simulink model "AWFG_concept_Phase1"  (R2018a)
settings: Solver=ode3  StartTime=0.0  StopTime=0.1  RelTol=1e-3  EnableMultiTasking=on
libraries: simulink x7
Description:
  | AWFG_concept: This model explores the implementation concept
  | of an arbitrary waveform generator (AWFG) in a real-time target
  | platform with a combination of CPU and FPGA code.
  | This concepts aims at minimizing changes in the FPGA programming.
settings Model: Creator=Estra  LastModifiedBy=Talha Rao
settings DataIOCC: LimitDataPoints=on  SaveFormat=Array
settings OptimizationCC: DefaultParameterBehavior=Inlined  UseDivisionForNetSlopeComputation=on  UseFloatMulNetSlope=on  InlineInvariantSignals=on  PassReuseOutputArgsAs=Individual arguments  ExpressionDepthLimit=2147483647  ZeroExternalMemoryAtStartup=off  ZeroInternalMemoryAtStartup=off  NoFixptDivByZeroProtection=on  EfficientFloat2IntCast=on  LifeSpan=1
settings DebuggingCC: SignalInfNanChecking=warning  UnderspecifiedInitializationDetection=Classic  MergeDetectMultiDrivingBlocksExec=none  SolverPrmCheckMsg=warning  ParameterTunabilityLossMsg=error  UniqueDataStoreMsg=warning  AllowSymbolicDim=off  StateNameClashWarn=warning  SFUnexpectedBacktrackingDiag=warning  SFNoUnconditionalDefaultTransitionDiag=warning  SFExecutionAtInitializationDiag=none
settings HardwareCC: ProdLongLongMode=on
settings ModelReferenceCC: PropagateSignalLabelsOutOfModel=off
settings SFSimCC: MATLABDynamicMemAlloc=off
settings RTWCC: SystemTargetFile=ert.tlc  TemplateMakefile=ert_default_tmf  GenerateReport=on  IncludeHyperlinkInReport=on  LaunchReport=on  GenerateTraceInfo=on  GenerateTraceReport=on  GenerateTraceReportSl=on  GenerateTraceReportSf=on  GenerateTraceReportEml=on  GenerateCodeMetricsReport=on
settings CodeAppCC: ForceParamTrailComments=on  IgnoreCustomStorageClasses=off  OperatorAnnotations=on  SimulinkDataObjDesc=on  SFDataObjDesc=on  CustomSymbolStrGlobalVar=rt$N$M  CustomSymbolStrType=$N$M  CustomSymbolStrFcn=$N$M$F  CustomSymbolStrMacro=$N$M  InsertBlockDesc=on  StateflowObjectComments=on
settings ERTTargetCC: GenerateSampleERTMain=on  IncludeMdlTerminateFcn=off  CombineSignalStateStructs=on  SupportAbsoluteTime=off  SupportComplex=off  SupportNonInlinedSFcns=on  InlinedParameterPlacement=NonHierarchical  ERTCustomFileTemplate=example_file_process.tlc  ERTFilePackagingFormat=CompactWithDataFile
settings ConfigComp: CovMetricSettings=dw  CovHtmlReporting=on  CovSaveCumulativeToWorkspaceVar=on  CovSaveSingleToWorkspaceVar=on  CovExternalEMLEnable=off

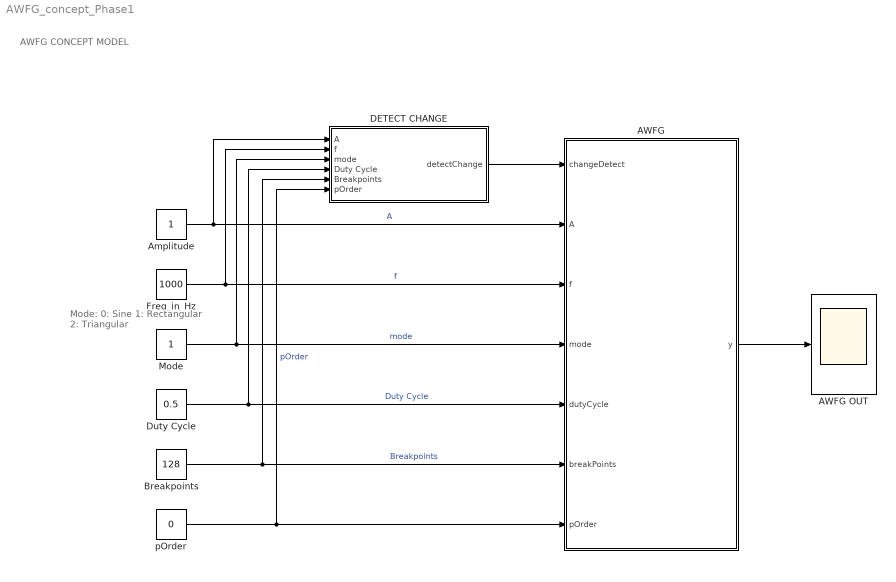
== system AWFG_concept_Phase1 ==
  note: AWFG CONCEPT MODEL
  note: Mode:
      | 0: Sine
      | 1: Rectangular
      | 2: Triangular
  AWFG : Subsystem
  AWFG OUT : Scope
  Amplitude : Constant
  Breakpoints : Constant  Value=128
  DETECT CHANGE : Subsystem
  Duty Cycle : Constant  Value=0.5
  Freq_in_Hz : Constant  Value=1000
  Mode : Constant
  pOrder : Constant  Value=0
  wires:
  AWFG/1(y) -> AWFG OUT/1
  DETECT CHANGE/1(detectChange) -> AWFG/1(changeDetect)
  Amplitude/1 -> DETECT CHANGE/1(A), AWFG/2(A)  "A"
  Freq_in_Hz/1 -> DETECT CHANGE/2(f), AWFG/3(f)  "f"
  Mode/1 -> DETECT CHANGE/3(mode), AWFG/4(mode)  "mode"
  Duty Cycle/1 -> DETECT CHANGE/4(Duty Cycle), AWFG/5(dutyCycle)  "Duty Cycle"
  Breakpoints/1 -> DETECT CHANGE/5(Breakpoints), AWFG/6(breakPoints)  "Breakpoints"
  pOrder/1 -> DETECT CHANGE/6(pOrder), AWFG/7(pOrder)  "pOrder"

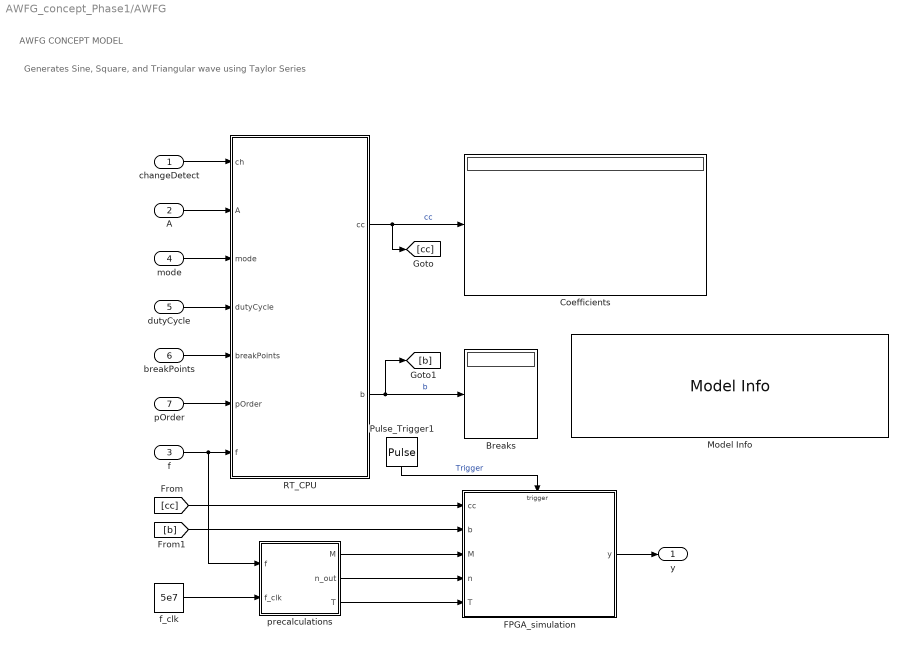
== system AWFG_concept_Phase1/AWFG ==
  note: Generates Sine, Square, and Triangular wave using Taylor Series
  note: AWFG CONCEPT MODEL
  changeDetect : Inport
  A : Inport  Port=2
  f : Inport  Port=3
  mode : Inport  Port=4
  dutyCycle : Inport  Port=5
  breakPoints : Inport  Port=6
  pOrder : Inport  Port=7
  Breaks : Display
  Coefficients : Display
  FPGA_simulation : Subsystem
  Model Info : simulink/Model-Wide Utilities/Model Info  Frame=on  DisplayStringWithTags=|  HorizontalTextAlignment=Left  LeftAlignmentValue=0.02
      | Model Info
      | Creator:       R. Estrada, FH JOANNEUM, 2018
      | Modified by: %<ModifiedBy>
      | Modify Date: %<ModifiedDate>
      | Version:%<ModelVersion>
      | Description:
      | %<Description>
  Pulse_Trigger1 : DiscretePulseGenerator  PulseType=Time based  Period=1/5e7  PulseWidth=50
  RT_CPU : MATLAB Function  TreatAsAtomicUnit=on
  f_clk : Constant  Value=5e7
  precalculations : Subsystem
  y : Outport
  wires:
  RT_CPU/2(b) -> [b], Breaks/1  "b"
  f_clk/1 -> precalculations/2(f_clk)
  RT_CPU/1(cc) -> Coefficients/1, [cc]  "cc"
  mode/1 -> RT_CPU/3(mode)
  f/1 -> precalculations/1(f), RT_CPU/7(f)
  breakPoints/1 -> RT_CPU/5(breakPoints)
  precalculations/2(n_out) -> FPGA_simulation/4(n)
  Pulse_Trigger1/1 -> FPGA_simulation/Trigger  "Trigger"
  precalculations/1(M) -> FPGA_simulation/3(M)
  precalculations/3(T) -> FPGA_simulation/5(T)
  FPGA_simulation/1(y) -> y/1
  A/1 -> RT_CPU/2(A)
  pOrder/1 -> RT_CPU/6(pOrder)
  dutyCycle/1 -> RT_CPU/4(dutyCycle)
  changeDetect/1 -> RT_CPU/1(ch)
  [b] -> FPGA_simulation/2(b)
  [cc] -> FPGA_simulation/1(cc)

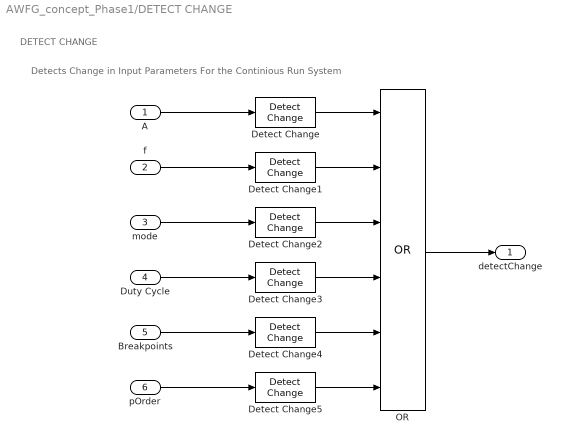
== system AWFG_concept_Phase1/DETECT CHANGE ==
  note: Detects Change in Input Parameters For the Continious Run System
  note: DETECT CHANGE
  A : Inport
  f : Inport  Port=2
  mode : Inport  Port=3
  Duty Cycle : Inport  Port=4
  Breakpoints : Inport  Port=5
  pOrder : Inport  Port=6
  Detect Change{,1..5} (6 alike) : simulink/Logic and Bit Operations/Detect Change  vinit=0  OutDataTypeStr=boolean
  OR : Logic  Operator=OR  Inputs=6  AllPortsSameDT=off  OutDataTypeStr=boolean
  detectChange : Outport
  wires:
  Detect Change3/1 -> OR/4
  mode/1 -> Detect Change2/1
  Detect Change5/1 -> OR/6
  Detect Change1/1 -> OR/2
  Breakpoints/1 -> Detect Change4/1
  pOrder/1 -> Detect Change5/1
  Detect Change4/1 -> OR/5
  Detect Change2/1 -> OR/3
  Detect Change/1 -> OR/1
  Duty Cycle/1 -> Detect Change3/1
  f/1 -> Detect Change1/1
  A/1 -> Detect Change/1
  OR/1 -> detectChange/1

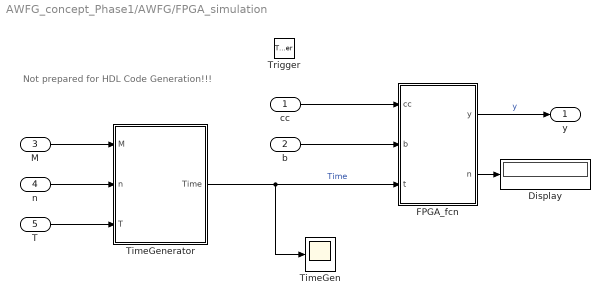
== system AWFG_concept_Phase1/AWFG/FPGA_simulation ==
  note: Not prepared for HDL Code Generation!!!
  cc : Inport
  b : Inport  Port=2
  M : Inport  Port=3
  n : Inport  Port=4
  T : Inport  Port=5
  Trigger : TriggerPort  VariantControl=(inherit)  PortDimensions=1
  Display : Display
  FPGA_fcn : MATLAB Function  TreatAsAtomicUnit=on
  TimeGen : Scope
  TimeGenerator : Subsystem
  y : Outport
  wires:
  T/1 -> TimeGenerator/3(T)
  n/1 -> TimeGenerator/2(n)
  cc/1 -> FPGA_fcn/1(cc)
  M/1 -> TimeGenerator/1(M)
  TimeGenerator/1(Time) -> FPGA_fcn/3(t), TimeGen/1  "Time"
  FPGA_fcn/1(y) -> y/1  "y"
  b/1 -> FPGA_fcn/2(b)
  FPGA_fcn/2(n) -> Display/1

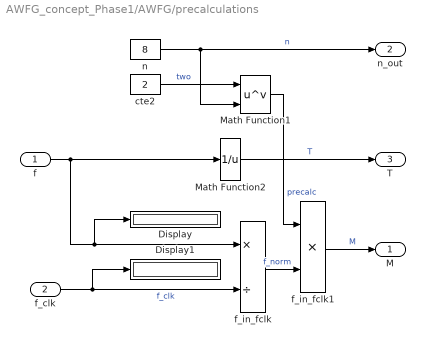
== system AWFG_concept_Phase1/AWFG/precalculations ==
  f : Inport
  f_clk : Inport  Port=2
  Display : Display
  Display1 : Display
  Math Function1 : Math  Operator=pow  SaturateOnIntegerOverflow=on
  Math Function2 : Math  Operator=reciprocal  SaturateOnIntegerOverflow=on
  cte2 : Constant  Value=2  SampleTime=-1
  f_in_fclk : Product  Inputs=*/
  f_in_fclk1 : Product  Inputs=**
  n : Constant  Value=8  SampleTime=-1
  M : Outport
  n_out : Outport  Port=2
  T : Outport  Port=3
  wires:
  cte2/1 -> Math Function1/1  "two"
  n/1 -> Math Function1/2, n_out/1  "n"
  Math Function1/1 -> f_in_fclk1/1  "precalc"
  Math Function2/1 -> T/1  "T"
  f_in_fclk1/1 -> M/1  "M"
  f_clk/1 -> f_in_fclk/2, Display1/1  "f_clk"
  f_in_fclk/1 -> f_in_fclk1/2  "f_norm"
  f/1 -> Math Function2/1, Display/1, f_in_fclk/1

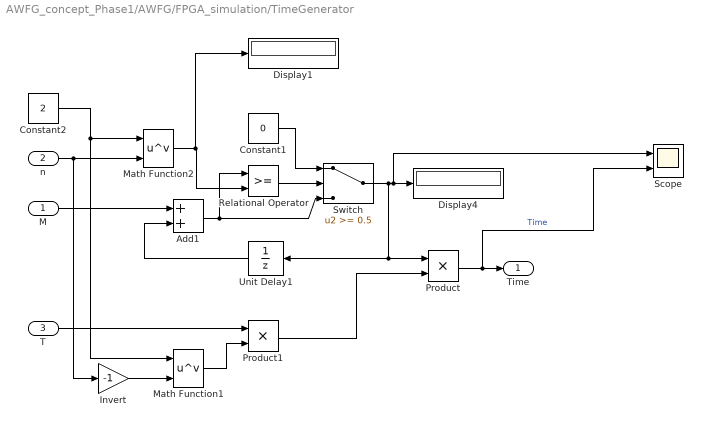
== system AWFG_concept_Phase1/AWFG/FPGA_simulation/TimeGenerator ==
  M : Inport
  n : Inport  Port=2
  T : Inport  Port=3
  Add1 : Sum
  Constant1 : Constant  Value=0
  Constant2 : Constant  Value=2
  Display1 : Display
  Display4 : Display
  Invert : Gain  Gain=-1
  Math Function1 : Math  Operator=pow  SaturateOnIntegerOverflow=on
  Math Function2 : Math  Operator=pow  SaturateOnIntegerOverflow=on
  Product : Product
  Product1 : Product
  Relational Operator : RelationalOperator  OutDataTypeStr=boolean  RndMeth=Nearest
  Scope : Scope  NumInputPorts=2
  Switch : Switch  Threshold=0.5
  Unit Delay1 : UnitDelay  SampleTime=-1
  Time : Outport
  wires:
  T/1 -> Product1/1
  Invert/1 -> Math Function1/2
  Constant2/1 -> Math Function1/1, Math Function2/1
  n/1 -> Math Function2/2, Invert/1
  Math Function2/1 -> Relational Operator/2, Display1/1
  Math Function1/1 -> Product1/2
  Product/1 -> Scope/2, Time/1  "Time"
  Product1/1 -> Product/2
  Switch/1 -> Unit Delay1/1, Product/1, Scope/1, Display4/1
  Unit Delay1/1 -> Add1/2
  M/1 -> Add1/1
  Constant1/1 -> Switch/1
  Relational Operator/1 -> Switch/2
  Add1/1 -> Switch/3, Relational Operator/1

== matlab function AWFG_concept_Phase1/AWFG/FPGA_simulation/FPGA_fcn ==
  data: y output; cc input; b input; t input; n output
function [y,n]  = fcn(cc,b,t)
%% FPGA_simulation
%   This Embedded Matlab function solves a 4th-order polynomial output 
%       according to the coefficients and breaks points given as input. 
%
%
%       NOTE: In the final implementation this fcn will be placed at the    
%             FPGA
%       
%    Author: R. Estrada, FH JOANNEUM, 2018
%
%%

%#codegen

    n=size(cc,2)-1;
    i=find(b>t,1);       % find closest upper break point
    ii=max(i(1)-1,1);    % assign actual index for polynomial calculation

    % Calculate polynomial output according to actual relative time
    y=0;
    for j=0:1:n                
        y=y+cc(ii,j+1)*(t-b(ii))^j;
    end

end

== matlab function AWFG_concept_Phase1/AWFG/RT_CPU ==
  data: ch input; A input [0..1]; mode input [0..2]; dutyCycle input [0..1]; breakPoints input [4..255]; pOrder input [0..3]; f input [0..10000]; cc output size=[256 4]; b output size=[1 255] [4..255]
function [cc,b]  = fcn(ch,A,mode,dutyCycle, breakPoints,pOrder, f)
%% RT CPU
%   This Embedded Matlab function calculates the polynomial coefficients
%       and breaks points according to the external user settings. 
%       Three different waveforms can be selected with "mode"
%               0: Sine
%               1: Rectangular (not implemented yet)
%               2: Triangular  (not implemented yet)
%
%       
%    Author: R. Estrada, FH JOANNEUM, 2018
%
%%
    % Declaration of global variables
    persistent cc0 b0 i0;
    % This is executed only once during Initialization
    if isempty(cc0)    
        cc0 = zeros(101,3);
        b0  = zeros(1,101);
        i0  = 0;  %Used to checks if the program is running for the 1st time
    end
    if (ch || i0<1)        
        
        i0=1;
        ch = 0;
        
        %Bound values of breakpoints
        assert(breakPoints<=256);
        
        cc = zeros(breakPoints+1,3);        %% Creates coefficients array 
        b  = zeros(1,(breakPoints + 1));    %% Create breakpoints array 
        tf = 1/f;
        y  = zeros(1 , (breakPoints + 1));

        
        switch mode
            case 0 % Sine wave
                                
                y  = A*sin(2*pi.*linspace(0,1,breakPoints+1));   
            
            case 1 % Square Wave 
 
                x= linspace(0,1,breakPoints+1);
                y = (x < dutyCycle).*(A) + (x >= dutyCycle).*(-A);
                y(breakPoints+1) = A;
                    
            case 2 % Triangular wave

                x= linspace(0,1,breakPoints +1);
                x1= linspace(0,1,breakPoints);
                
                if (dutyCycle ==0 || dutyCycle == 1)     %To avoid division by 0
                    
                    y = (dutyCycle == 1).*(-A+(x1*A*2)) +...
                        (dutyCycle ==0).*(-A+((1-x1)*A*2));
                    y= [y y(1)];
                else
                    
                    y = (x <= dutyCycle).*(-A+(x*A*(2/dutyCycle)))+...
                        (x > dutyCycle).*(-A+((1-x)*A*(2/(1-dutyCycle))));

                end
               
            otherwise
                y  = [0 0 0 0 0];
        end

        %% Finite difference
        %   Coefficients
        cfd = [  1 0 0 0;...
                -1 1 0 0; ...
                 1 -2 1 0; ...
                -1 3 -3 1];

        % Extend array around the end
        yy = [y y(2:4)];
        
        for j=0:1:breakPoints                        % Sweep of break points
            b(1,j+1)=j*tf/breakPoints;               % Store actual break point
            ys = [yy(j+1) yy(j+2) yy(j+3) yy(j+4)];   % Prepare y vector
            for i=0:1:pOrder       
                dy = cfd(i+1,:) * ys'/(tf/breakPoints)^i; % Compute pOrder derivate        
                cc(j+1,i+1)= dy/factorial(i);        
            end                  
        end
        
        % Store values in global variables
        cc0 = cc;  
        b0  = b;
    else
        % Keep the previous values
        cc = cc0;
        b  = b0;
    end %end of main if
    
end % Function
